simulink library "datacenterCompositeLib"  (R2025b)
settings: Solver=VariableStepAuto  StartTime=0.0  StopTime=10.0  RelTol=1e-3
undefined symbols (not defined in the file): DiscIntNeverNeededParam, ee_sli_rtmsupport, gcbh, Ts, ups
libraries: fl_lib x129, datacenter_lib x32, nesl_utility x16, $bdroot x14, SimscapeFluids_lib x8, simulink x8, eeGeneralControl x6, ee_lib x4, eeTransforms x4, slpidlib x3, eeSinusoidalMeasurementV2 x2, simulink_extras x1
(part 3 of 5)

== system datacenterCompositeLib/PDU Racks (TL) ==
  FMamb : datacenter_lib/Flow Multiplier
      settings: InternalSimscapePortConfiguration="{\"Bottom\":[],\"Left\":[{\"id\":\"A\",\"label\":\"A\",\"type\":\"foundation.thermal_liquid.thermal_liquid\"}],\"Right\":[{\"id\":\"B\",\"label\":\"B\",\"type\":\"foundation.thermal_liquid.thermal_liquid\"}],\"Top\":[{\"id\":\"Na\",\"label\":\"Na\",\"type\":\"input\"},{\"id\":\"Nb\",\"label\":\"Nb\",\"type\":\"input\"}]}"
  FMcdu : datacenter_lib/Flow Multiplier
      settings: InternalSimscapePortConfiguration="{\"Bottom\":[],\"Left\":[{\"id\":\"A\",\"label\":\"A\",\"type\":\"foundation.thermal_liquid.thermal_liquid\"}],\"Right\":[{\"id\":\"B\",\"label\":\"B\",\"type\":\"foundation.thermal_liquid.thermal_liquid\"}],\"Top\":[{\"id\":\"Na\",\"label\":\"Na\",\"type\":\"input\"},{\"id\":\"Nb\",\"label\":\"Nb\",\"type\":\"input\"}]}"
  PS Product : fl_lib/Physical Signals/Functions/PS Product
  Server Tray (TL) : $bdroot/Server Tray (TL)  nGPU=nGPU  gpuTDPperDie=gpuTDPperDie  gpuIdlePower=gpuIdlePower  gpuHBMpower=gpuHBMpower  gpuExponent=gpuExponent  gpuHBMutil=gpuHBMutil  gpuLeakage=gpuLeakage  gpuNominalDieT=gpuNominalDieT  gpuDieThermalC=gpuDieThermalC  gpuHeatSinkR=gpuHeatSinkR  gpuSurfArea=gpuSurfArea  gpuAmbientR=gpuAmbientR  nCPU=nCPU  cpuTDPperSocket=cpuTDPperSocket  cpuIdlePower=cpuIdlePower  cpuExponent=cpuExponent  cpuLeakage=cpuLeakage  cpuNominalDieT=cpuNominalDieT  cpuDieThermalC=cpuDieThermalC  cpuHeatSinkR=cpuHeatSinkR  cpuSurfArea=cpuSurfArea  cpuAmbientR=cpuAmbientR  trayMass=trayMass  trayCp=trayCp  trayThermalR=trayThermalR  pipeLen=pipeLen  pipeArea=pipeArea  pipeDia=pipeDia  pipeLenXtra=pipeLenXtra  thermalKtc=thermalKtc  initialT=initialT  initialP=initialP  htc=htc
  TMamb : datacenter_lib/Thermal Multiplier
      settings: InternalSimscapePortConfiguration="{\"Bottom\":[],\"Left\":[{\"id\":\"A\",\"label\":\"A\",\"type\":\"foundation.thermal.thermal\"}],\"Right\":[{\"id\":\"B\",\"label\":\"B\",\"type\":\"foundation.thermal.thermal\"}],\"Top\":[{\"id\":\"Na\",\"label\":\"Na\",\"type\":\"input\"},{\"id\":\"Nb\",\"label\":\"Nb\",\"type\":\"input\"}]}"
  nTraysXnRacks : fl_lib/Physical Signals/Sources/PS Constant  constant=nTrays*nRacks
  one : fl_lib/Physical Signals/Sources/PS Constant  constant=1
  U_gpu : PMIOPort  Side=Left
  U_cpu : PMIOPort  Port=2  Side=Left
  Ha : PMIOPort  Port=3  Side=Left
  P : PMIOPort  Port=4  Side=Right
  T_gpu : PMIOPort  Port=5  Side=Right
  T_cpu : PMIOPort  Port=6  Side=Right
  A : PMIOPort  Port=7  Side=Right
  B : PMIOPort  Port=8  Side=Right
  connections:
  Server Tray (TL)/RConn1 -- PS Product/LConn2
  Server Tray (TL)/LConn2 -- U_cpu/RConn1
  Server Tray (TL)/RConn3 -- T_cpu/RConn1
  Server Tray (TL)/RConn2 -- T_gpu/RConn1
  FMcdu/LConn1 -- Server Tray (TL)/RConn5
  FMamb/LConn1 -- Server Tray (TL)/RConn4
  PS Product/LConn1 -- TMamb/LConn3 -- FMcdu/LConn2 -- FMamb/LConn2 -- nTraysXnRacks/RConn1
  FMamb/LConn3 -- FMcdu/LConn3 -- TMamb/LConn2 -- one/RConn1
  FMcdu/RConn1 -- B/RConn1
  FMamb/RConn1 -- A/RConn1
  PS Product/RConn1 -- P/RConn1
  Server Tray (TL)/LConn1 -- U_gpu/RConn1
  TMamb/RConn1 -- Server Tray (TL)/LConn3
  TMamb/LConn1 -- Ha/RConn1

== system datacenterCompositeLib/Rack Air Cooling ==
  Flowrate vs Eff : fl_lib/Physical Signals/Lookup Tables/PS Lookup Table (1D)  x=flowVec m^3/s  f=fanEffVec  interp_method=simscape.enum.interpolation.linear  extrap_method=simscape.enum.extrapolation.nearest
  Flowrate vs Pressure Drop : fl_lib/Physical Signals/Lookup Tables/PS Lookup Table (1D)  x=flowVec m^3/s  f=prDropVec Pa  interp_method=simscape.enum.interpolation.linear  extrap_method=simscape.enum.extrapolation.nearest
  MaxFlowrate : fl_lib/Physical Signals/Functions/PS Gain  gain=max(flowVec) m^3/s
  PS Divide : fl_lib/Physical Signals/Functions/PS Divide
  PS Product : fl_lib/Physical Signals/Functions/PS Product
  PS Product1 : fl_lib/Physical Signals/Functions/PS Product
  PS Saturation : fl_lib/Physical Signals/Nonlinear Operators/PS Saturation  upper_limit=1  lower_limit=0  ZeroCross=true
  Q : Subsystem
  dT : Subsystem
      settings: PortSchema="{\"entries\":[{\"content\":{\"sides\":[{\"content\":{\"connectorIds\":[\"LConn1\"]},\"type\":\"ConnectorPlacement.EquallySpacedRectSide\",\"uuid\":\"24179a54-9ef9-408d-b9e3-71fcbe48c3e7\"},{\"content\":{\"connectorIds\":[\"RConn1\"],\"side\":\"RIGHT\"},\"type\":\"ConnectorPlacement.EquallySpacedRectSide\",\"uuid\":\"9ef8b705-2d29-4693-9aa8-2fb03fb72ba0\"},{\"content\":{\"side\":\"TOP\"},\"type\":\"ConnectorPlacement.EquallySpacedRectSide\",\"uuid\":\"67fd6558-0b74-41b6-9065-c50d20bb7de5\"},{\"content\":{\"connectorIds\":[\"RConn2\"],\"side\":\"BOTTOM\"},\"type\":\"ConnectorPlacement.EquallySpacedRectSide\",\"uuid\":\"dead0843-c913-4c5f-8840-2a92db603c86\"}]},\"type\":\"ConnectorPlacement.EquallySpacedConnector\",\"uuid\":\"734a32c8-d564-4672-86f6-d3d1b9b4eb6d\"}],\"packageUris\":[\"http://schema.mathworks.com/mf0/Connector/R2020b\"],\"version\":\"1.0\"}"
  m_dot_Cp : Subsystem
      settings: PortSchema="{\"entries\":[{\"content\":{\"sides\":[{\"content\":{},\"type\":\"ConnectorPlacement.EquallySpacedRectSide\",\"uuid\":\"30dae9bf-ed85-460d-bbc0-602f54b59459\"},{\"content\":{\"side\":\"RIGHT\"},\"type\":\"ConnectorPlacement.EquallySpacedRectSide\",\"uuid\":\"05907a20-db7b-437b-af9c-28a9e12dbb0f\"},{\"content\":{\"connectorIds\":[\"LConn1\"],\"side\":\"TOP\"},\"type\":\"ConnectorPlacement.EquallySpacedRectSide\",\"uuid\":\"1394250d-0f3a-4d32-aa79-d5be723ed221\"},{\"content\":{\"connectorIds\":[\"RConn1\"],\"side\":\"BOTTOM\"},\"type\":\"ConnectorPlacement.EquallySpacedRectSide\",\"uuid\":\"8d71629e-6ed3-4a45-8875-f0ad6e4187c2\"}]},\"type\":\"ConnectorPlacement.EquallySpacedConnector\",\"uuid\":\"77e9989b-961e-42ca-a28b-c98959ddb965\"}],\"packageUris\":[\"http://schema.mathworks.com/mf0/Connector/R2020b\"],\"version\":\"1.0\"}"
  numFans : fl_lib/Physical Signals/Sources/PS Constant  constant=nFans
  C : PMIOPort  Side=Left
  S : PMIOPort  Port=2  Side=Left
  H : PMIOPort  Port=3  Side=Right
  P : PMIOPort  Port=4  Side=Right
  connections:
  Flowrate vs Eff/LConn1 -- PS Product/LConn2 -- Flowrate vs Pressure Drop/LConn1 -- MaxFlowrate/RConn1 -- m_dot_Cp/RConn1
  PS Product1/LConn2 -- PS Product/RConn1
  PS Saturation/LConn1 -- S/RConn1
  PS Product1/RConn1 -- PS Divide/LConn1
  PS Divide/LConn2 -- Flowrate vs Eff/RConn1
  PS Divide/RConn1 -- P/RConn1
  PS Saturation/RConn1 -- MaxFlowrate/LConn1
  numFans/RConn1 -- PS Product1/LConn1
  PS Product/LConn1 -- Flowrate vs Pressure Drop/RConn1
  Q/RConn1 -- dT/RConn1 -- H/RConn1
  dT/LConn1 -- C/RConn1
  Q/LConn1 -- dT/RConn2
  m_dot_Cp/LConn1 -- Q/LConn2

== system datacenterCompositeLib/Server Tray ==
  AmbCPU : fl_lib/Thermal/Thermal Elements/Convective Heat Transfer  thermal_type=foundation.enum.constant_variable.constant  area=cpuSurfArea*nCPU m^2  heat_tr_coeff=htc W/(K*m^2)  min_heat_tr_coeff=1e-3 W/(K*m^2)  T_specify=off  T_priority=None  T=0 K  T_nominal_specify=off  T_nominal_value=1  T_nominal_unit=K  Q_specify=off  Q_priority=None  Q=0 W  Q_nominal_specify=off  Q_nominal_value=1  Q_nominal_unit=W
  AmbGPU : fl_lib/Thermal/Thermal Elements/Convective Heat Transfer  thermal_type=foundation.enum.constant_variable.constant  area=gpuSurfArea*nGPU m^2  heat_tr_coeff=htc W/(K*m^2)  min_heat_tr_coeff=1e-3 W/(K*m^2)  T_specify=off  T_priority=None  T=0 K  T_nominal_specify=off  T_nominal_value=1  T_nominal_unit=K  Q_specify=off  Q_priority=None  Q=0 W  Q_nominal_specify=off  Q_nominal_value=1  Q_nominal_unit=W
  PS Add : fl_lib/Physical Signals/Functions/PS Add
  Server Chip CPU : datacenter_lib/Server Chip  processorType=ProcessorType.CPU  numGPUs=4  numCPUs=nCPU  gpuTDP=1200 W  gpuIdlePower=300 W  gpuPowerExponent=1.4  hbmPowPerGPU=80 W  hbmUtilizationFrac=0.7  cpuTDP=cpuTDPperSocket W  cpuIdlePower=cpuIdlePower W  cpuPowerExponent=cpuExponent  PleakageCoeff=cpuLeakage W/K  chipTnominal=cpuNominalDieT K  chipCth=cpuDieThermalC J/K  T_specify=on  T_priority=High  T=initialT K  T_nominal_specify=off  T_nominal_value=1  T_nominal_unit=K  Q_specify=off  Q_priority=None  Q=0 W  Q_nominal_specify=off  Q_nominal_value=1  Q_nominal_unit=W
      settings: InternalSimscapePortConfiguration="{\"Bottom\":[{\"id\":\"H\",\"label\":\"H\",\"type\":\"foundation.thermal.thermal\"}],\"Left\":[{\"id\":\"U\",\"label\":\"U\",\"type\":\"input\"}],\"Right\":[{\"id\":\"Pow\",\"label\":\"P\",\"type\":\"output\"},{\"id\":\"Tchip\",\"label\":\"T\",\"type\":\"output\"}],\"Top\":[]}"
  Server Chip GPU : datacenter_lib/Server Chip  processorType=ProcessorType.GPU  numGPUs=nGPU  numCPUs=nCPU  gpuTDP=gpuTDPperDie W  gpuIdlePower=gpuIdlePower W  gpuPowerExponent=gpuExponent  hbmPowPerGPU=gpuHBMpower W  hbmUtilizationFrac=gpuHBMutil  cpuTDP=cpuTDPperSocket W  cpuIdlePower=cpuIdlePower W  cpuPowerExponent=1.1  PleakageCoeff=gpuLeakage W/K  chipTnominal=gpuNominalDieT K  chipCth=gpuDieThermalC J/K  T_specify=on  T_priority=High  T=initialT K  T_nominal_specify=off  T_nominal_value=1  T_nominal_unit=K  Q_specify=off  Q_priority=None  Q=0 W  Q_nominal_specify=off  Q_nominal_value=1  Q_nominal_unit=W
      settings: InternalSimscapePortConfiguration="{\"Bottom\":[{\"id\":\"H\",\"label\":\"H\",\"type\":\"foundation.thermal.thermal\"}],\"Left\":[{\"id\":\"U\",\"label\":\"U\",\"type\":\"input\"}],\"Right\":[{\"id\":\"Pow\",\"label\":\"P\",\"type\":\"output\"},{\"id\":\"Tchip\",\"label\":\"T\",\"type\":\"output\"}],\"Top\":[]}"
  TR_CPU_Amb : fl_lib/Thermal/Thermal Elements/Thermal Resistance  resistance=cpuAmbientR/nGPU K/W  T_specify=off  T_priority=None  T=0 K  T_nominal_specify=off  T_nominal_value=1  T_nominal_unit=K  Q_specify=off  Q_priority=None  Q=0 W  Q_nominal_specify=off  Q_nominal_value=1  Q_nominal_unit=W
  TR_CPU_substrate : fl_lib/Thermal/Thermal Elements/Thermal Resistance  resistance=cpuHeatSinkR/nGPU K/W  T_specify=off  T_priority=None  T=0 K  T_nominal_specify=off  T_nominal_value=1  T_nominal_unit=K  Q_specify=off  Q_priority=None  Q=0 W  Q_nominal_specify=off  Q_nominal_value=1  Q_nominal_unit=W
  TR_GPU_Amb : fl_lib/Thermal/Thermal Elements/Thermal Resistance  resistance=gpuAmbientR/nGPU K/W  T_specify=off  T_priority=None  T=0 K  T_nominal_specify=off  T_nominal_value=1  T_nominal_unit=K  Q_specify=off  Q_priority=None  Q=0 W  Q_nominal_specify=off  Q_nominal_value=1  Q_nominal_unit=W
  TR_GPU_substrate : fl_lib/Thermal/Thermal Elements/Thermal Resistance  resistance=gpuHeatSinkR/nGPU K/W  T_specify=off  T_priority=None  T=0 K  T_nominal_specify=off  T_nominal_value=1  T_nominal_unit=K  Q_specify=off  Q_priority=None  Q=0 W  Q_nominal_specify=off  Q_nominal_value=1  Q_nominal_unit=W
  TR_Tray_Amb : fl_lib/Thermal/Thermal Elements/Thermal Resistance  resistance=trayThermalR K/W  T_specify=off  T_priority=None  T=0 K  T_nominal_specify=off  T_nominal_value=1  T_nominal_unit=K  Q_specify=off  Q_priority=None  Q=0 W  Q_nominal_specify=off  Q_nominal_value=1  Q_nominal_unit=W
  Tray Thermal Mass : fl_lib/Thermal/Thermal Elements/Thermal Mass  mass_type=foundation.enum.constant_variable.constant  mass=trayMass kg  sp_heat=trayCp J/(K*kg)  mass_min=1e-6 kg  num_ports=foundation.enum.numPorts2.two  m_specify=off  m_priority=High  m=1 kg  m_nominal_specify=off  m_nominal_value=1  m_nominal_unit=kg  T_specify=on  T_priority=High  T=initialT K  T_nominal_specify=off  T_nominal_value=1  T_nominal_unit=K  Q_specify=off  Q_priority=None  Q=0 W  Q_nominal_specify=off  Q_nominal_value=1  Q_nominal_unit=W
      settings: InternalSimscapePortConfiguration="{\"Bottom\":[],\"Left\":[{\"id\":\"M\",\"label\":\"\",\"type\":\"foundation.thermal.thermal\"}],\"Right\":[{\"id\":\"N\",\"label\":\"\",\"type\":\"foundation.thermal.thermal\"}],\"Top\":[]}"
  U_gpu : PMIOPort  Side=Left
  U_cpu : PMIOPort  Port=2  Side=Left
  P : PMIOPort  Port=3  Side=Right
  T_gpu : PMIOPort  Port=4  Side=Right
  T_cpu : PMIOPort  Port=5  Side=Right
  Hc : PMIOPort  Port=6  Side=Right
  Ha : PMIOPort  Port=7  Side=Left
  connections:
  Tray Thermal Mass/LConn1 -- TR_GPU_substrate/RConn1 -- TR_CPU_substrate/RConn1
  Server Chip GPU/RConn2 -- T_gpu/RConn1
  TR_CPU_substrate/LConn1 -- TR_CPU_Amb/LConn1 -- Server Chip CPU/RConn3
  TR_GPU_Amb/RConn1 -- Server Chip GPU/RConn3 -- TR_GPU_substrate/LConn1
  TR_Tray_Amb/LConn1 -- Tray Thermal Mass/RConn1
  Server Chip GPU/LConn1 -- U_gpu/RConn1
  Server Chip CPU/LConn1 -- U_cpu/RConn1
  Server Chip CPU/RConn2 -- T_cpu/RConn1
  TR_Tray_Amb/RConn1 -- Hc/RConn1
  AmbGPU/LConn1 -- TR_GPU_Amb/LConn1
  AmbCPU/RConn1 -- AmbGPU/RConn1 -- Ha/RConn1
  P/RConn1 -- PS Add/RConn1
  PS Add/LConn1 -- Server Chip GPU/RConn1
  PS Add/LConn2 -- Server Chip CPU/RConn1
  AmbCPU/LConn1 -- TR_CPU_Amb/RConn1

== system datacenterCompositeLib/Server Tray (TL) ==
  Cold Plate : $bdroot/Cold Plate  pipeLen=pipeLen  pipeArea=pipeArea  pipeDia=pipeDia  pipeLenXtra=pipeLenXtra  thermalR=thermalKtc  initialT=initialT  initialP=initialP
  Server Tray : $bdroot/Server Tray  nGPU=nGPU  gpuTDPperDie=gpuTDPperDie  gpuIdlePower=gpuIdlePower  gpuHBMpower=gpuHBMpower  gpuExponent=gpuExponent  gpuHBMutil=gpuHBMutil  gpuLeakage=gpuLeakage  gpuNominalDieT=gpuNominalDieT  gpuDieThermalC=gpuDieThermalC  gpuHeatSinkR=gpuHeatSinkR  gpuSurfArea=gpuSurfArea  gpuAmbientR=gpuAmbientR  nCPU=nCPU  cpuTDPperSocket=cpuTDPperSocket  cpuIdlePower=cpuIdlePower  cpuExponent=cpuExponent  cpuLeakage=cpuLeakage  cpuNominalDieT=cpuNominalDieT  cpuDieThermalC=cpuDieThermalC  cpuHeatSinkR=cpuHeatSinkR  cpuSurfArea=cpuSurfArea  cpuAmbientR=cpuAmbientR  trayMass=trayMass  trayCp=trayCp  trayThermalR=trayThermalR  initialT=initialT  htc=htc
  U_gpu : PMIOPort  Side=Left
  U_cpu : PMIOPort  Port=2  Side=Left
  Ha : PMIOPort  Port=3  Side=Left
  P : PMIOPort  Port=4  Side=Right
  T_gpu : PMIOPort  Port=5  Side=Right
  T_cpu : PMIOPort  Port=6  Side=Right
  A : PMIOPort  Port=7  Side=Right
  B : PMIOPort  Port=8  Side=Right
  connections:
  Cold Plate/LConn2 -- Server Tray/RConn4
  Server Tray/LConn3 -- Ha/RConn1
  Server Tray/LConn1 -- U_gpu/RConn1
  Server Tray/LConn2 -- U_cpu/RConn1
  Cold Plate/LConn1 -- A/RConn1
  Cold Plate/RConn1 -- B/RConn1
  Server Tray/RConn1 -- P/RConn1
  Server Tray/RConn3 -- T_cpu/RConn1
  Server Tray/RConn2 -- T_gpu/RConn1

== system datacenterCompositeLib/Solid State Transformer ==
  note: Cascaded H-Bridge modules with DAB
  note: DAB Control
  note: Rectifier Control
  Constant1 : Constant  Value=dcBusVoltage
  Constant2 : Constant  Value=0
  Converters : Subsystem
      settings: PortSchema="{\"entries\":[{\"content\":{\"sides\":[{\"content\":{\"connectorIds\":[\"In1\",\"In2\",\"LConn1\"]},\"type\":\"ConnectorPlacement.EquallySpacedRectSide\",\"uuid\":\"3c50ecae-d327-4517-ac35-d4ccad8214d6\"},{\"content\":{\"connectorIds\":[\"RConn1\",\"RConn2\",\"Out1\",\"Out2\"],\"side\":\"RIGHT\"},\"type\":\"ConnectorPlacement.EquallySpacedRectSide\",\"uuid\":\"ce483151-8cc4-4e89-a036-44eb982feae5\"},{\"content\":{\"side\":\"TOP\"},\"type\":\"ConnectorPlacement.EquallySpacedRectSide\",\"uuid\":\"39146706-ffb9-4bd3-97cb-72551c78d2ac\"}]},\"type\":\"ConnectorPlacement.EquallySpacedConnector\",\"uuid\":\"8cf16702-94fc-4b9b-91c9-b502d0239b3b\"}],\"packageUris\":[\"http://schema.mathworks.com/mf0/Connector/R2020b\"],\"version\":\"1.0\"}"
  DAB Controller : Subsystem
  DC Voltage Balancing : Subsystem
  Filter & AC measurements : Subsystem
  PFC Rectifier Controller : Subsystem  LoadFcn=%ee_sli_rtmsupport( 'loadfcn', gcbh );  mask(PFC Rectifier Controller (Three-Phase)){Freq=60, L=0.01, BaseImpedance=9.522, KpPLL=15, KiPLL=100, Ts=5e-05, KpVoltage=18, KiVoltage=500, KdVoltage=0, NdVoltage=100, BaseVdc=4400, VoltControlUpperLimit=1, VoltControlLowerLimit=-1, KpdCurrent=10, KidCurrent=200, KddCurrent=0, IdControlUpperLimit=1, IdControlLowerLimit=-1, KpqCurrent=10, KiqCurrent=200, KdqCurrent=0, NdCurrent=100, IqControlUpperLimit=1, IqControlLowerLimit=-1}
      mask prompts: Freq "physmod:ee:library:comments:control:eeConverterControllers:SystemFrequencyHz_MP"; L "physmod:ee:library:comments:control:eeConverterControllers:ACFilterInductanceH_MP"; BaseImpedance "physmod:ee:library:comments:control:eeConverterControllers:ACSideBaseImpedanceOhm_MP"; KpPLL "physmod:ee:library:comments:control:eeConverterControllers:PLLProportionalGain_MP"; KiPLL "physmod:ee:library:comments:control:eeConverterControllers:PLLIntegralGain_MP"; Ts "physmod:ee:library:comments:control:eeConverterControllers:SampleTime1ForInherited_MP"; KpVoltage "physmod:ee:library:comments:control:eeConverterControllers:ProportionalGain_MP"; KiVoltage "physmod:ee:library:comments:control:eeConverterControllers:IntegralGain_MP"; KdVoltage "physmod:ee:library:comments:control:eeConverterControllers:DerivativeGain_MP"; NdVoltage "physmod:ee:library:comments:control:eeConverterControllers:DerivativeControllerFilterCoefficientN_MP"; BaseVdc "physmod:ee:library:comments:control:eeConverterControllers:DCBusBaseVoltageV_MP"; VoltControlUpperLimit "physmod:ee:library:comments:control:eeConverterControllers:ControllerOutputUpperLimitpu_MP"; VoltControlLowerLimit "physmod:ee:library:comments:control:eeConverterControllers:ControllerOutputLowerLimitpu_MP"; KpdCurrent "physmod:ee:library:comments:control:eeConverterControllers:IdProportionalGain_MP"; KidCurrent "physmod:ee:library:comments:control:eeConverterControllers:IdIntegralGain_MP"; KddCurrent "physmod:ee:library:comments:control:eeConverterControllers:IdDerivativeGain_MP"; IdControlUpperLimit "physmod:ee:library:comments:control:eeConverterControllers:IdControllerOutputUpperLimitpu_MP"; IdControlLowerLimit "physmod:ee:library:comments:control:eeConverterControllers:IdControllerOutputLowerLimitpu_MP"; KpqCurrent "physmod:ee:library:comments:control:eeConverterControllers:IqProportionalGain_MP"; KiqCurrent "physmod:ee:library:comments:control:eeConverterControllers:IqIntegralGain_MP"; KdqCurrent "physmod:ee:library:comments:control:eeConverterControllers:IqDerivativeGain_MP"; NdCurrent "physmod:ee:library:comments:control:eeConverterControllers:DerivativeCurrentControllerFilterCoefficientN_MP"; IqControlUpperLimit "physmod:ee:library:comments:control:eeConverterControllers:IqControllerOutputUpperLimitpu_MP"; IqControlLowerLimit "physmod:ee:library:comments:control:eeConverterControllers:IqControllerOutputLowerLimitpu_MP"
      mask help: physmod:ee:library:comments:control:eeConverterControllers:PFCRectifierController_MD
      mask init:
      | ee.mask.initializePFCController(gcb,Ts, Freq, L,BaseImpedance,KpPLL,KiPLL,KpVoltage,KiVoltage,KdVoltage,BaseVdc, NdVoltage,VoltControlUpperLimit,VoltControlLowerLimit,KpdCurrent, KidCurrent, KddCurrent, NdCurrent, IdControlUpperLimit, IdControlLowerLimit, KpqCurrent, KiqCurrent, KdqCurrent, IqControlUpperLimit, IqControlLowerLimit);
      settings: CopyFcn=%ee_sli_rtmsupport( 'copyfcn', gcbh );  DeleteFcn=ee_sli_rtmsupport( 'deletefcn', gcbh );  ModelCloseFcn=ee_sli_rtmsupport( 'modelclosefcn', gcbh );  PostSaveFcn=ee_sli_rtmsupport( 'postsavefcn', gcbh );  PreCopyFcn=ee_sli_rtmsupport( 'precopyfcn', gcbh );  OpenFcn=ee_sli_rtmsupport( 'openfcn', gcbh );  CloseFcn=%ee_sli_rtmsupport( 'closefcn', gcbh );  PreDeleteFcn=ee_sli_rtmsupport( 'predeletefcn', gcbh );
      mask Help: web(nesl_help(gcbh))
      mask DialogControl GeneralTabVal Prompt: physmod:ee:library:comments:control:eeConverterControllers:tab_General
      mask DialogControl Freq Prompt: System frequency (Hz)
      mask DialogControl L Prompt: AC filter inductance (H)
      mask DialogControl BaseImpedance Prompt: AC side base impedance (Ohm)
      mask DialogControl KpPLL Prompt: PLL proportional gain
      mask DialogControl KiPLL Prompt: PLL integral gain
      mask DialogControl Ts Prompt: Sample time (-1 for inherited)
      mask DialogControl VoltageControl Prompt: physmod:ee:library:comments:control:eeConverterControllers:tab_VoltageController
      mask DialogControl KpVoltage Prompt: Proportional gain
      mask DialogControl KiVoltage Prompt: Integral gain
      mask DialogControl KdVoltage Prompt: Derivative gain
      mask DialogControl NdVoltage Prompt: Derivative controller filter coefficient (N)
      mask DialogControl BaseVdc Prompt: DC bus base voltage (V)
      mask DialogControl VoltControlUpperLimit Prompt: Controller output upper limit (pu)
      mask DialogControl VoltControlLowerLimit Prompt: Controller output lower limit (pu)
      mask DialogControl CurrentControl Prompt: physmod:ee:library:comments:control:eeConverterControllers:tab_CurrentController
      mask DialogControl KpdCurrent Prompt: Id proportional gain
      mask DialogControl KidCurrent Prompt: Id integral gain
      mask DialogControl KddCurrent Prompt: Id derivative gain
      mask DialogControl IdControlUpperLimit Prompt: Id controller output upper limit (pu)
      mask DialogControl IdControlLowerLimit Prompt: Id controller output lower limit (pu)
      mask DialogControl KpqCurrent Prompt: Iq proportional gain
      mask DialogControl KiqCurrent Prompt: Iq integral gain
      mask DialogControl KdqCurrent Prompt: Iq derivative gain
      mask DialogControl NdCurrent Prompt: Derivative current controller filter coefficient (N)
      mask DialogControl IqControlUpperLimit Prompt: Iq controller output upper limit (pu)
      mask DialogControl IqControlLowerLimit Prompt: Iq controller output lower limit (pu)
  + : PMIOPort  Side=Right
  - : PMIOPort  Port=2  Side=Right
  ABC : PMIOPort  Port=3  Side=Left
  Out1 : Outport
  wires:
  Constant2/1 -> PFC Rectifier Controller/2(QRef (pu))
  Constant1/1 -> PFC Rectifier Controller/1(VdcRef (V))
  Filter & AC measurements/1(Vabc) -> PFC Rectifier Controller/4(VabcSens (pu))
  Converters/2(VdcMeas) -> PFC Rectifier Controller/3(VdcSens (V))
  Filter & AC measurements/2(Iabc) -> PFC Rectifier Controller/5(IabcSens (pu))
  DC Voltage Balancing/1(mabc) -> Converters/1(mabc)
  Converters/1(Vdc) -> DAB Controller/1(Vdc), DC Voltage Balancing/1(Vdc)
  DAB Controller/1(phi) -> Converters/2(phi)
  PFC Rectifier Controller/1(VabcRef (pu)) -> DC Voltage Balancing/2(VabcRef)
  PFC Rectifier Controller/2(Visualization) -> DAB Controller/2(Vac)
  PFC Rectifier Controller/3(Flag) -> Out1/1
  connections:
  Filter & AC measurements/LConn1 -- ABC/RConn1
  -/RConn1 -- Converters/RConn2
  +/RConn1 -- Converters/RConn1
  Filter & AC measurements/RConn1 -- Converters/LConn1

== system datacenterCompositeLib/CDU (LUT)/flowrate ==
  PS Product2 : fl_lib/Physical Signals/Functions/PS Product
  PS Saturation : fl_lib/Physical Signals/Nonlinear Operators/PS Saturation  upper_limit=speed  lower_limit=0  ZeroCross=true
  PS Subtract : fl_lib/Physical Signals/Functions/PS Subtract
  flowrate : fl_lib/Physical Signals/Functions/PS Add
  max_flowrate : fl_lib/Physical Signals/Sources/PS Constant  constant=max(flowrate_vec) m^3/s
  min_flowrate : fl_lib/Physical Signals/Sources/PS Constant  constant=min(flowrate_vec) m^3/s
  S : PMIOPort  Side=Left
  F : PMIOPort  Port=2  Side=Right
  connections:
  max_flowrate/RConn1 -- PS Subtract/LConn1
  PS Saturation/RConn1 -- PS Product2/LConn2
  PS Subtract/RConn1 -- PS Product2/LConn1
  flowrate/RConn1 -- F/RConn1
  min_flowrate/RConn1 -- PS Subtract/LConn2 -- flowrate/LConn2
  flowrate/LConn1 -- PS Product2/RConn1
  S/RConn1 -- PS Saturation/LConn1

== system datacenterCompositeLib/CDU (TL)/Pump Efficiency ==
  PS Abs : fl_lib/Physical Signals/Nonlinear Operators/PS Abs  ZeroCross=true
      settings: InternalSimscapePortConfiguration="{\"Bottom\":[],\"Left\":[{\"id\":\"I\",\"label\":\"\",\"type\":\"input\"}],\"Right\":[{\"id\":\"O\",\"label\":\"\",\"type\":\"output\"}],\"Top\":[]}"
  PS Abs1 : fl_lib/Physical Signals/Nonlinear Operators/PS Abs  ZeroCross=true
      settings: InternalSimscapePortConfiguration="{\"Bottom\":[],\"Left\":[{\"id\":\"I\",\"label\":\"\",\"type\":\"input\"}],\"Right\":[{\"id\":\"O\",\"label\":\"\",\"type\":\"output\"}],\"Top\":[]}"
  PS Abs2 : fl_lib/Physical Signals/Nonlinear Operators/PS Abs  ZeroCross=true
      settings: InternalSimscapePortConfiguration="{\"Bottom\":[],\"Left\":[{\"id\":\"I\",\"label\":\"\",\"type\":\"input\"}],\"Right\":[{\"id\":\"O\",\"label\":\"\",\"type\":\"output\"}],\"Top\":[]}"
  PS Product1 : fl_lib/Physical Signals/Functions/PS Product
  Pump Eff. : fl_lib/Physical Signals/Lookup Tables/PS Lookup Table (1D)  x=pumpCapacityVec m^3/s  f=pumpEff  interp_method=simscape.enum.interpolation.linear  extrap_method=simscape.enum.extrapolation.nearest
  ePower : fl_lib/Physical Signals/Functions/PS Divide
  nPump : fl_lib/Physical Signals/Functions/PS Divide
  P : PMIOPort  Side=Left
  V : PMIOPort  Port=2  Side=Left
  E : PMIOPort  Port=3  Side=Right
  N : PMIOPort  Port=4  Side=Left
  connections:
  ePower/LConn1 -- PS Abs/RConn1
  Pump Eff./RConn1 -- ePower/LConn2
  P/RConn1 -- PS Product1/LConn2
  PS Abs/LConn1 -- PS Product1/RConn1
  V/RConn1 -- nPump/LConn1 -- PS Product1/LConn1
  nPump/LConn2 -- N/RConn1
  PS Abs1/LConn1 -- ePower/RConn1
  PS Abs1/RConn1 -- E/RConn1
  PS Abs2/RConn1 -- Pump Eff./LConn1
  PS Abs2/LConn1 -- nPump/RConn1

== system datacenterCompositeLib/CDU (TL)/Subsystem ==
  Ideal Angular Velocity Source : fl_lib/Mechanical/Mechanical Sources/Ideal Angular Velocity Source
  Ideal Torque Sensor : fl_lib/Mechanical/Mechanical Sensors/Ideal Torque Sensor
  Mechanical Rotational Reference : fl_lib/Mechanical/Rotational Elements/Mechanical Rotational Reference
  R : PMIOPort  Side=Left
  C : PMIOPort  Port=2  Side=Left
  rpm : PMIOPort  Port=3  Side=Right
  connections:
  Ideal Angular Velocity Source/LConn1 -- Ideal Torque Sensor/LConn1
  rpm/RConn1 -- Ideal Angular Velocity Source/RConn1
  R/RConn1 -- Ideal Torque Sensor/RConn1
  Mechanical Rotational Reference/LConn1 -- C/RConn1 -- Ideal Angular Velocity Source/RConn2

== system datacenterCompositeLib/Rack Air Cooling/Q ==
  Controlled Heat Flow Rate Source : fl_lib/Thermal/Thermal Sources/Controlled Heat Flow Rate Source
  PS Product2 : fl_lib/Physical Signals/Functions/PS Product
  Thermal Reference : fl_lib/Thermal/Thermal Elements/Thermal Reference
  dT : PMIOPort  Side=Left
  m.Cp : PMIOPort  Port=2  Side=Left
  Q : PMIOPort  Port=3  Side=Right
  connections:
  PS Product2/RConn1 -- Controlled Heat Flow Rate Source/RConn1
  Thermal Reference/LConn1 -- Controlled Heat Flow Rate Source/RConn2
  PS Product2/LConn1 -- dT/RConn1
  Controlled Heat Flow Rate Source/LConn1 -- Q/RConn1
  m.Cp/RConn1 -- PS Product2/LConn2

== system datacenterCompositeLib/Rack Air Cooling/dT ==
  Cold : fl_lib/Thermal/Thermal Sensors/Temperature Sensor  temperature_measure=foundation.enum.MeasurementReference.absolute
      settings: InternalSimscapePortConfiguration="{\"Bottom\":[],\"Left\":[{\"id\":\"A\",\"label\":\"A\",\"type\":\"foundation.thermal.thermal\"}],\"Right\":[{\"id\":\"T\",\"label\":\"T\",\"type\":\"output\"}],\"Top\":[]}"
  Hot : fl_lib/Thermal/Thermal Sensors/Temperature Sensor  temperature_measure=foundation.enum.MeasurementReference.absolute
      settings: InternalSimscapePortConfiguration="{\"Bottom\":[],\"Left\":[{\"id\":\"A\",\"label\":\"A\",\"type\":\"foundation.thermal.thermal\"}],\"Right\":[{\"id\":\"T\",\"label\":\"T\",\"type\":\"output\"}],\"Top\":[]}"
  PS Subtract : fl_lib/Physical Signals/Functions/PS Subtract
  C : PMIOPort  Side=Left
  H : PMIOPort  Port=2  Side=Right
  dT : PMIOPort  Port=3  Side=Right
  connections:
  Cold/LConn1 -- C/RConn1
  dT/RConn1 -- PS Subtract/RConn1
  PS Subtract/LConn1 -- Cold/RConn1
  PS Subtract/LConn2 -- Hot/RConn1
  Hot/LConn1 -- H/RConn1

== system datacenterCompositeLib/Rack Air Cooling/m_dot_Cp ==
  Fluid Density : fl_lib/Physical Signals/Sources/PS Constant  constant=fluidDen kg/m^3
  Fluid Sp. Heat : fl_lib/Physical Signals/Sources/PS Constant  constant=fluidCp J/(K*kg)
  PS Product3 : fl_lib/Physical Signals/Functions/PS Product
  PS Product4 : fl_lib/Physical Signals/Functions/PS Product
  " " : PMIOPort  Side=Left
  m : PMIOPort  Port=2  Side=Right
  connections:
  PS Product4/LConn2 -- PS Product3/RConn1
  Fluid Density/RConn1 -- PS Product3/LConn1
  PS Product3/LConn2 -- m/RConn1
  PS Product4/LConn1 -- Fluid Sp. Heat/RConn1
  PS Product4/RConn1 -- " "/RConn1

== system datacenterCompositeLib/Solid State Transformer/Converters ==
  note: DAB Phase shift signal
  note: Reference signal for H-Bridge
  mabc : Inport
  phi : Inport  Port=2
  Add : Sum  Inputs=+++
  Add1 : Sum  Inputs=+++
  Bus Creator : BusCreator  Inputs=5
  Demux : Demux  Outputs=3
  Demux1 : Demux  Outputs=3
  Electrical Reference1 : fl_lib/Electrical/Electrical Elements/Electrical Reference
  Gain_1_1 : Gain  Gain=1/3
  Gain_1_3 : Gain  Gain=1/3
  Phase Splitter : ee_lib/Connectors & References/Phase Splitter
  Subsystem1 : Subsystem
  Subsystem2 : Subsystem
  Subsystem3 : Subsystem
  ABC2 : PMIOPort  Side=Left
  + : PMIOPort  Port=2  Side=Right
  - : PMIOPort  Port=3  Side=Right
  Vdc : Outport
  VdcMeas : Outport  Port=2
  wires:
  Subsystem1/1(Out1) -> Bus Creator/1, Add/1  "AVdc"
  Subsystem2/1(Out1) -> Add/2, Bus Creator/2  "BAVdc"
  Subsystem3/1(Out1) -> Bus Creator/3, Add/3  "CVdc"
  Add/1 -> Gain_1_3/1
  Gain_1_3/1 -> VdcMeas/1, Bus Creator/4  "AvGVdc"
  Bus Creator/1 -> Vdc/1
  phi/1 -> Demux1/1
  Subsystem2/2(V_out_pu) -> Add1/2
  Subsystem1/2(V_out_pu) -> Add1/1
  Subsystem3/2(V_out_pu) -> Add1/3
  Add1/1 -> Gain_1_1/1
  Gain_1_1/1 -> Bus Creator/5  "PUVdc"
  Demux1/1 -> Subsystem1/1(PhA)
  Demux1/2 -> Subsystem2/1(PhB)
  Demux1/3 -> Subsystem3/1(PhC)
  mabc/1 -> Demux/1
  Demux/1 -> Subsystem1/2(ma)
  Demux/2 -> Subsystem2/2(mb)
  Demux/3 -> Subsystem3/2(mc)
  connections:
  Subsystem1/LConn2 -- Subsystem2/LConn2 -- Subsystem3/LConn2 -- Electrical Reference1/LConn1
  Subsystem3/LConn1 -- Phase Splitter/RConn3
  Subsystem1/LConn1 -- Phase Splitter/RConn1
  Subsystem1/RConn2 -- Subsystem3/RConn2 -- -/RConn1 -- Subsystem2/RConn2
  Subsystem2/LConn1 -- Phase Splitter/RConn2
  Subsystem1/RConn1 -- Subsystem3/RConn1 -- Subsystem2/RConn1 -- +/RConn1
  Phase Splitter/LConn1 -- ABC2/RConn1

== system datacenterCompositeLib/Solid State Transformer/DAB Controller ==
  Vdc : Inport
  Vac : Inport  Port=2
  AND_gate : Logic  AllPortsSameDT=off  OutDataTypeStr=boolean
  AND_reset : Logic  AllPortsSameDT=off  OutDataTypeStr=boolean
  Add : Sum
  Add1 : Sum
  Add2 : Sum
  Bus Selector : BusSelector  OutputSignals=AVdc,BAVdc,CVdc,AvGVdc,PUVdc
  Bus Selector1 : BusSelector  OutputSignals=pllVmag [pu],reset
  Constant : Constant  Value=0
  DAB Balancing : Subsystem
  Error : Sum  Inputs=+-
  Mux : Mux  Inputs=3
  Mux1 : Mux  Inputs=3
  PI_central : slpidlib/PID Controller  Controller=PI  Form=Parallel  TimeDomain=Discrete-time  UseExternalTs=off  SampleTime=5e-05  IntegratorMethod=Forward Euler  FilterMethod=Forward Euler  ControllerParametersSource=internal  P=5.5  I=130  UseKiTs=off  D=0  UseExternalDerivativeSource=off  N=100  UseFilter=on  TunerSelectOption=Transfer Function Based (PID Tuner App)  InitialConditionSource=internal  InitialConditionForIntegrator=0  InitialConditionForFilter=0  DifferentiatorICPrevScaledInput=0  ExternalReset=falling  TrackingMode=off  Kt=1  LimitOutput=on  SatLimitsSource=internal  UpperSaturationLimit=0.45  LowerSaturationLimit=-0.45  LinearizeAsGain=off  AntiWindupMode=none  Kb=1  LimitIntegrator=off  UpperIntegratorSaturationLimit=inf  LowerIntegratorSaturationLimit=-inf  POutMin=[]  POutMax=[]  IOutMin=[]  IOutMax=[]  DOutMin=[]  DOutMax=[]  NOutMin=[]  NOutMax=[]  SumOutMin=[]  SumOutMax=[]  SaturationOutMin=[]  SaturationOutMax=[]  PParamMin=[]  PParamMax=[]  IParamMin=[]  IParamMax=[]  DParamMin=[]  DParamMax=[]  NParamMin=[]  NParamMax=[]  KbParamMin=[]  KbParamMax=[]  KtParamMin=[]  KtParamMax=[]  KbOutMin=[]  KbOutMax=[]  KtOutMin=[]  KtOutMax=[]  IntegratorOutMin=[]  IntegratorOutMax=[]  FilterOutMin=[]  FilterOutMax=[]  SumI1OutMin=[]  SumI1OutMax=[]  SumI2OutMin=[]  SumI2OutMax=[]  SumI3OutMin=[]  SumI3OutMax=[]  SumI4OutMin=[]  SumI4OutMax=[]  SumDOutMin=[]  SumDOutMax=[]  DifferentiatorOutMin=[]  DifferentiatorOutMax=[]  FilterDiffOutCoefMin=[]  FilterDiffOutCoefMax=[]  ReciprocalOutMin=[]  ReciprocalOutMax=[]  SumDenOutMin=[]  SumDenOutMax=[]  SumNumOutMin=[]  SumNumOutMax=[]  DivideOutMin=[]  DivideOutMax=[]  UdiffTsProdOutMin=[]  UdiffTsProdOutMax=[]  NTsProdOutMin=[]  NTsProdOutMax=[]  UintegralTsProdOutMin=[]  UintegralTsProdOutMax=[]  UngainTsProdOutMin=[]  UngainTsProdOutMax=[]  ClampingZeroOutDataTypeStr=Inherit: Inherit via back propagation  ClampingZeroOutMin=[]  ClampingZeroOutMax=[]  FilterDenConstantOutDataTypeStr=Inherit: Inherit via back propagation  FilterDenConstantOutMin=[]  FilterDenConstantOutMax=[]  PCopyOutDataTypeStr=Inherit: Inherit via back propagation  PCopyOutMin=[]  PCopyOutMax=[]  NCopyOutDataTypeStr=Inherit: Inherit via back propagation  NCopyOutMin=[]  NCopyOutMax=[]  IntegratorContinuousStateAttributes=''  IntegratorStateMustResolveToSignalObject=off  IntegratorRTWStateStorageClass=Auto  FilterContinuousStateAttributes=''  FilterStateMustResolveToSignalObject=off  FilterRTWStateStorageClass=Auto  ParallelPVariant=InternalParameters  IdealPVariant=Disabled  IVariant=InternalParameters  DVariant=Disabled  IntegratorVariant=Discrete  SatVariant=Enabled  AWVariant=Passthrough  PCopyVariant=Disabled  TRVariant=Disabled  FdbkBlocksVariant=Forward  IdealPFdbkVariant=Disabled  SatFdbkVariant=Disabled  DerivativeFilterVariant=Disabled  NVariant=Disabled  NCopyVariant=Disabled_SignalSpec  FilterICVariant=Disabled  IntegratorICVariant=InternalICs  ExternalResetVariant=ExternalReset  TRSumVariant=Passthrough  SumFdbkVariant=Disabled  SumVariant=Sum_PI  TsampFilterVariant=InternalTs  TsampNgainVariant=Passthrough  TsampIntegralVariant=Disabled_SignalSpec  ExternalSaturationOutDataTypeStr=Inherit: Same as second input  DerivativeSourceVariant=Disabled  PreIntVariant=InternalPreInt
      settings: LibrarySourceBlock=simulink/Discrete/Discrete PID Controller
  StartupDelay : Step  SampleTime=0
  Switch : Switch  Criteria=u2 > Threshold  SaturateOnIntegerOverflow=off  InputSameDT=off
  VacLowRelay : Relay  OnSwitchValue=0.48  OffSwitchValue=0.42  OnOutputValue=0  OffOutputValue=1
  Vref : Constant
  phi : Outport
  wires:
  Vref/1 -> Error/1
  Error/1 -> PI_central/1
  PI_central/1 -> Add1/1, Add2/1, Add/1
  Vdc/1 -> Bus Selector/1
  Bus Selector/1 -> DAB Balancing/1(Vdc_A)  "<AVdc>"
  Bus Selector/2 -> DAB Balancing/2(Vdc_B)  "<BAVdc>"
  Bus Selector/3 -> DAB Balancing/3(Vdc_C)  "<CVdc>"
  Bus Selector/4 -> DAB Balancing/4(Vdc_avg)  "<AvGVdc>"
  Bus Selector/5 -> Error/2  "<PUVdc>"
  DAB Balancing/1(delta_d_A) -> Add/2  "delta_d_A"
  DAB Balancing/2(delta_d_B) -> Add1/2  "delta_d_B"
  DAB Balancing/3(delta_d_C) -> Add2/2  "delta_d_C"
  Add/1 -> Mux/1
  Add2/1 -> Mux/3
  Add1/1 -> Mux/2
  Mux/1 -> Switch/3
  Vac/1 -> Bus Selector1/1
  Bus Selector1/1 -> VacLowRelay/1  "<pllVmag [pu]>"
  Switch/1 -> phi/1
  Constant/1 -> Mux1/3, Mux1/2, Mux1/1
  Mux1/1 -> Switch/1
  StartupDelay/1 -> AND_gate/2, AND_reset/2
  AND_gate/1 -> Switch/2
  Bus Selector1/2 -> AND_reset/1  "<reset>"
  AND_reset/1 -> PI_central/2
  VacLowRelay/1 -> AND_gate/1

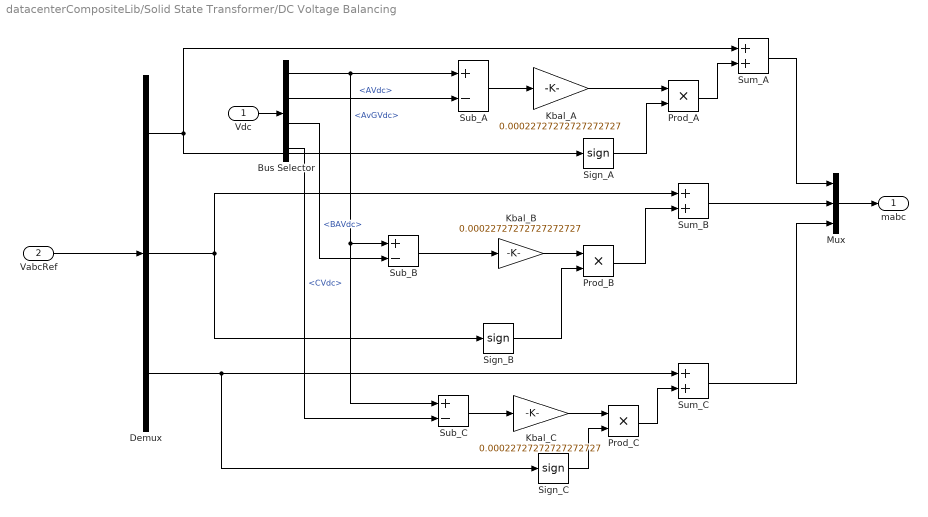
== system datacenterCompositeLib/Solid State Transformer/DC Voltage Balancing ==
  Vdc : Inport
  VabcRef : Inport  Port=2
  Bus Selector : BusSelector  OutputSignals=AvGVdc,AVdc,BAVdc,CVdc
  Demux : Demux  Outputs=3
  Kbal_A : Gain  Gain=0.00022727272727272727
  Kbal_B : Gain  Gain=0.00022727272727272727
  Kbal_C : Gain  Gain=0.00022727272727272727
  Mux : Mux  Inputs=3
  Prod_A : Product
  Prod_B : Product
  Prod_C : Product
  Sign_A : Signum
  Sign_B : Signum
  Sign_C : Signum
  Sub_A : Sum  Inputs=+-
  Sub_B : Sum  Inputs=+-
  Sub_C : Sum  Inputs=+-
  Sum_A : Sum
  Sum_B : Sum
  Sum_C : Sum
  mabc : Outport
  wires:
  Sub_B/1 -> Kbal_B/1
  Prod_B/1 -> Sum_B/2
  Sub_A/1 -> Kbal_A/1
  Sub_C/1 -> Kbal_C/1
  Kbal_A/1 -> Prod_A/1
  Sign_A/1 -> Prod_A/2
  Kbal_C/1 -> Prod_C/1
  Sign_C/1 -> Prod_C/2
  Kbal_B/1 -> Prod_B/1
  Sign_B/1 -> Prod_B/2
  Prod_A/1 -> Sum_A/2
  Prod_C/1 -> Sum_C/2
  Bus Selector/1 -> Sub_C/1, Sub_B/1, Sub_A/1  "<AvGVdc>"
  VabcRef/1 -> Demux/1
  Demux/1 -> Sum_A/1, Sign_A/1
  Demux/2 -> Sum_B/1, Sign_B/1
  Demux/3 -> Sign_C/1, Sum_C/1
  Sum_B/1 -> Mux/2
  Sum_A/1 -> Mux/1
  Sum_C/1 -> Mux/3
  Mux/1 -> mabc/1
  Vdc/1 -> Bus Selector/1
  Bus Selector/2 -> Sub_A/2  "<AVdc>"
  Bus Selector/3 -> Sub_B/2  "<BAVdc>"
  Bus Selector/4 -> Sub_C/2  "<CVdc>"

== system datacenterCompositeLib/Solid State Transformer/Filter & AC measurements ==
  Current : Subsystem
  Current and Voltage Sensor (Three-Phase) : ee_lib/Sensors & Transducers/Current and Voltage Sensor (Three-Phase)  vMeasurementType=ee.enum.vmeasurement.lg  outputUnit=ee.enum.unit.pu  SRated=20e6 A*V  VRated=13800 V  I_specify=off  I_priority=None  I=[0, 0, 0] A  I_nominal_specify=off  I_nominal_value=1  I_nominal_unit=A  V_specify=off  V_priority=None  V=[0, 0, 0] V  V_nominal_specify=off  V_nominal_value=1  V_nominal_unit=V
      settings: InternalSimscapePortConfiguration="{\"Bottom\":[],\"Left\":[{\"id\":\"N1\",\"label\":\"~1\",\"type\":\"foundation.electrical.three_phase\"}],\"Right\":[{\"id\":\"V_output\",\"label\":\"V\",\"type\":\"output\"},{\"id\":\"I_output\",\"label\":\"I\",\"type\":\"output\"},{\"id\":\"N2\",\"label\":\"~2\",\"type\":\"foundation.electrical.three_phase\"}],\"Top\":[]}"
  Gain : Gain  Gain=1/(5e6)
  Gain1 : Gain  Gain=1/(5e6)
  Low-Pass Filter (Discrete or Continuous)1 : eeGeneralControl/Low-Pass Filter (Discrete or Continuous)  K=1  T=10e-3  B=inf  A=-inf  init_option=Inherited from block input  x0=0  Ts=-1
  Low-Pass Filter (Discrete or Continuous)2 : eeGeneralControl/Low-Pass Filter (Discrete or Continuous)  K=1  T=10e-3  B=inf  A=-inf  init_option=Inherited from block input  x0=0  Ts=-1
  PLL : Subsystem  Commented=on
      settings: PortSchema="{\"entries\":[{\"content\":{\"sides\":[{\"content\":{\"connectorIds\":[\"Out1\",\"Out2\",\"Out3\"]},\"type\":\"ConnectorPlacement.EquallySpacedRectSide\",\"uuid\":\"76485780-20fe-4fcf-8224-69648da6ed2a\"},{\"content\":{\"connectorIds\":[\"In1\",\"In2\"],\"side\":\"RIGHT\"},\"type\":\"ConnectorPlacement.EquallySpacedRectSide\",\"uuid\":\"f19a6390-e634-42c7-8d46-4cd80cbab182\"},{\"content\":{\"side\":\"TOP\"},\"type\":\"ConnectorPlacement.EquallySpacedRectSide\",\"uuid\":\"87682f72-1844-428e-be70-ad7ca3191ee3\"}]},\"type\":\"ConnectorPlacement.EquallySpacedConnector\",\"uuid\":\"f2136b07-48ec-402b-adb3-18c0bac2157c\"}],\"packageUris\":[\"http://schema.mathworks.com/mf0/Connector/R2020b\"],\"version\":\"1.0\"}"
  PS-Simulink Converter : nesl_utility/PS-Simulink Converter  PhysicalDomain=network_engine_domain  SubClassName=ps_output  LeftPortType=input  RightPortType=output  PseudoPeriodic=off  Frequencies=[]  VectorFormat=1-D array  Unit=inherit  AffineConversion=off
  PS-Simulink Converter1 : nesl_utility/PS-Simulink Converter  PhysicalDomain=network_engine_domain  SubClassName=ps_output  LeftPortType=input  RightPortType=output  PseudoPeriodic=off  Frequencies=[]  VectorFormat=1-D array  Unit=inherit  AffineConversion=off
  PS-Simulink Converter2 : nesl_utility/PS-Simulink Converter  PhysicalDomain=network_engine_domain  SubClassName=ps_output  LeftPortType=input  RightPortType=output  PseudoPeriodic=off  Frequencies=[]  VectorFormat=inherit  Unit=inherit  AffineConversion=off
  PS-Simulink Converter3 : nesl_utility/PS-Simulink Converter  PhysicalDomain=network_engine_domain  SubClassName=ps_output  LeftPortType=input  RightPortType=output  PseudoPeriodic=off  Frequencies=[]  VectorFormat=inherit  Unit=inherit  AffineConversion=off
  Power Sensor (Three-Phase) : ee_lib/Sensors & Transducers/Power Sensor (Three-Phase)  load_type=ee.enum.passive.type_balanced.balanced  f0=60 Hz
      settings: InternalSimscapePortConfiguration="{\"Bottom\":[],\"Left\":[{\"id\":\"N1\",\"label\":\"~1\",\"type\":\"foundation.electrical.three_phase\"}],\"Right\":[{\"id\":\"N2\",\"label\":\"~2\",\"type\":\"foundation.electrical.three_phase\"}],\"Top\":[{\"id\":\"Pm\",\"label\":\"P\",\"type\":\"output\"},{\"id\":\"Qm\",\"label\":\"Q\",\"type\":\"output\"}]}"
  RL filter : ee_lib/Passive/RLC Assemblies/RLC (Three-Phase)  port_option=ee.enum.threePhasePort.composite  component_structure=ee.enum.rlc.structure.SeriesRL  R=0.1 Ohm  L=0.01 H  C=1e-6 F  R_parasitic=1e-6 Ohm  G_parasitic=1e-6 1/Ohm  IL_specify=on  IL_priority=None  IL=[0, 0, 0] A  IL_nominal_specify=off  IL_nominal_value=1  IL_nominal_unit=A  VC_specify=on  VC_priority=None  VC=[0, 0, 0] V  VC_nominal_specify=off  VC_nominal_value=1  VC_nominal_unit=V
      settings: InternalSimscapePortConfiguration="{\"Bottom\":[],\"Left\":[{\"id\":\"N1\",\"label\":\"~1\",\"type\":\"foundation.electrical.three_phase\"}],\"Right\":[{\"id\":\"N2\",\"label\":\"~2\",\"type\":\"foundation.electrical.three_phase\"}],\"Top\":[]}"
  Terminator : Terminator
  Terminator1 : Terminator
  Voltage : Subsystem
  ABC : PMIOPort  Side=Left
  ABC2 : PMIOPort  Port=2  Side=Right
  Vabc : Outport
  Iabc : Outport  Port=2
  wires:
  PS-Simulink Converter/1 -> Current/1(Isabc)
  Current/1(Iabc) -> Iabc/1, PLL/1(Iabc)
  PS-Simulink Converter1/1 -> Voltage/1(Vsabc)
  Voltage/1(Vabc) -> Vabc/1, PLL/2(V)
  PS-Simulink Converter2/1 -> Gain/1
  PS-Simulink Converter3/1 -> Gain1/1
  Gain/1 -> Low-Pass Filter (Discrete or Continuous)1/1
  Gain1/1 -> Low-Pass Filter (Discrete or Continuous)2/1
  PLL/3(mag) -> ?
  PLL/2(freq) -> ?
  Low-Pass Filter (Discrete or Continuous)1/1 -> Terminator/1
  Low-Pass Filter (Discrete or Continuous)2/1 -> Terminator1/1
  connections:
  Current and Voltage Sensor (Three-Phase)/RConn2 -- PS-Simulink Converter/LConn1
  PS-Simulink Converter1/LConn1 -- Current and Voltage Sensor (Three-Phase)/RConn1
  Current and Voltage Sensor (Three-Phase)/LConn1 -- ABC/RConn1
  Power Sensor (Three-Phase)/RConn1 -- RL filter/LConn1
  Power Sensor (Three-Phase)/LConn2 -- PS-Simulink Converter2/LConn1
  Power Sensor (Three-Phase)/LConn3 -- PS-Simulink Converter3/LConn1
  RL filter/RConn1 -- ABC2/RConn1
  Power Sensor (Three-Phase)/LConn1 -- Current and Voltage Sensor (Three-Phase)/RConn3

== system datacenterCompositeLib/Solid State Transformer/PFC Rectifier Controller ==
  VdcRef (V) : Inport
  QRef (pu) : Inport  Port=2
  VdcSens (V) : Inport  Port=3
  VabcSens (pu) : Inport  Port=4
  IabcSens (pu) : Inport  Port=5
  Current Controller : Subsystem
  DC Voltage Controller and Current Reference : Subsystem
  PLL : Subsystem
      settings: PortSchema="{\"entries\":[{\"content\":{\"sides\":[{\"content\":{\"connectorIds\":[\"Out1\",\"Out2\",\"Out3\",\"Out4\"]},\"type\":\"ConnectorPlacement.EquallySpacedRectSide\",\"uuid\":\"76485780-20fe-4fcf-8224-69648da6ed2a\"},{\"content\":{\"connectorIds\":[\"In1\"],\"side\":\"RIGHT\"},\"type\":\"ConnectorPlacement.EquallySpacedRectSide\",\"uuid\":\"f19a6390-e634-42c7-8d46-4cd80cbab182\"},{\"content\":{\"side\":\"TOP\"},\"type\":\"ConnectorPlacement.EquallySpacedRectSide\",\"uuid\":\"87682f72-1844-428e-be70-ad7ca3191ee3\"}]},\"type\":\"ConnectorPlacement.EquallySpacedConnector\",\"uuid\":\"f2136b07-48ec-402b-adb3-18c0bac2157c\"}],\"packageUris\":[\"http://schema.mathworks.com/mf0/Connector/R2020b\"],\"version\":\"1.0\"}"
  Rate Transition : RateTransition  InitialCondition=1  OutPortSampleTime=Ts
  Reset Controller : Subsystem
  VabcRef (pu) : Outport
  Out Bus Element : Outport  Port=2  PortName=Visualization  Element=pllAngle [rad]
  Out Bus Element1 : Outport  Port=2  PortName=Visualization  Element=pllVmag [pu]
  Out Bus Element2 : Outport  Port=2  PortName=Visualization  Element=Idref [pu]
  Out Bus Element3 : Outport  Port=2  PortName=Visualization  Element=Iqref [pu]
  Out Bus Element5 : Outport  Port=2  PortName=Visualization  Element=IdCntrlError [pu]
  Out Bus Element6 : Outport  Port=2  PortName=Visualization  Element=IqCntrlError [pu]
  BusElementOut : Outport  Port=2  PortName=Visualization  Element=reset
  Flag : Outport  Port=3
  wires:
  Current Controller/3(IqCntrlError) -> Out Bus Element6/1
  Current Controller/2(IdCntrlError) -> Out Bus Element5/1
  PLL/1(theta) -> Out Bus Element/1, Current Controller/3(theta)
  Rate Transition/1 -> PLL/1(V)
  DC Voltage Controller and Current Reference/2(iqRef) -> Current Controller/2(iqRef), Out Bus Element3/1
  DC Voltage Controller and Current Reference/1(idRef) -> Out Bus Element2/1, Current Controller/1(idRef)
  IabcSens (pu)/1 -> Current Controller/6(iabc(PU))
  PLL/3(Vq) -> Current Controller/5(vq)
  VdcSens (V)/1 -> DC Voltage Controller and Current Reference/4(VdcSens)
  Current Controller/1(vabcRef) -> VabcRef (pu)/1
  PLL/4(mag) -> Current Controller/7(Vmag), Reset Controller/1(u), DC Voltage Controller and Current Reference/2(vPeak), Out Bus Element1/1
  QRef (pu)/1 -> DC Voltage Controller and Current Reference/1(qRef)
  VabcSens (pu)/1 -> Rate Transition/1
  VdcRef (V)/1 -> DC Voltage Controller and Current Reference/3(vdcRef)
  PLL/2(Vd) -> Current Controller/4(vd)
  Current Controller/4(Flag) -> Flag/1
  Reset Controller/1(Out1) -> Current Controller/8(Reset), BusElementOut/1, DC Voltage Controller and Current Reference/5(Reset)
